simulink model "Group10_Pacemaker_FinalSimulink"  (R2020a)
settings: Solver=FixedStepAuto  StartTime=0.0  StopTime=300  FixedStep=1e-3  RelTol=1e-3  EnableMultiTasking=on
undefined symbols (not defined in the file): a, A0, A1, b, c, D0, D1, D10, D11, D12, D13, D2, D3, D4, D5, D6, D7, D8, D9, PTA0, PTA1, PTA2, PTB2, PTB23, PTB3, PTB9, PTC16, PTC17, PTC2, PTC3, PTC4, PTD0, PTD1, PTD2, PTD3
libraries: frdmk64flib x23, etargetslib x20, simulink x2, dspstat3 x1, hdlsllib x1
settings Model: ExtModeTrigDuration=5  Creator=jilsh  LastModifiedBy=Priya Patel
settings OptimizationCC: EnhancedBackFolding=on  PassReuseOutputArgsAs=Individual arguments  ZeroExternalMemoryAtStartup=off  ZeroInternalMemoryAtStartup=off  MaxStackSize=64  OptimizeBlockOrder=speed  DifferentSizesBufferReuse=on  OptimizationCustomize=off  EfficientTunableParamExpr=on
settings DebuggingCC: ParameterTunabilityLossMsg=error  SFMachineParentedDataDiag=error
settings HardwareCC: ProdBitPerPointer=32  ProdBitPerSizeT=32  ProdBitPerPtrDiffT=32  ProdLargestAtomicInteger=Long  ProdLargestAtomicFloat=Double  ProdWordSize=32  ProdHWDeviceType=ARM Compatible->ARM Cortex
settings SFSimCC: MATLABDynamicMemAlloc=off
settings RTWCC: SystemTargetFile=ert.tlc  HardwareBoard=NXP FRDM-K64F  TemplateMakefile=ert_default_tmf  Toolchain=GNU Tools for ARM Embedded Processors
settings CodeAppCC: ForceParamTrailComments=on  IgnoreCustomStorageClasses=off  OperatorAnnotations=on  SimulinkDataObjDesc=on  SFDataObjDesc=on  InsertBlockDesc=on
settings ERTTargetCC: ExtModeTransport=4  ExtModeMexFile=sendToCommService

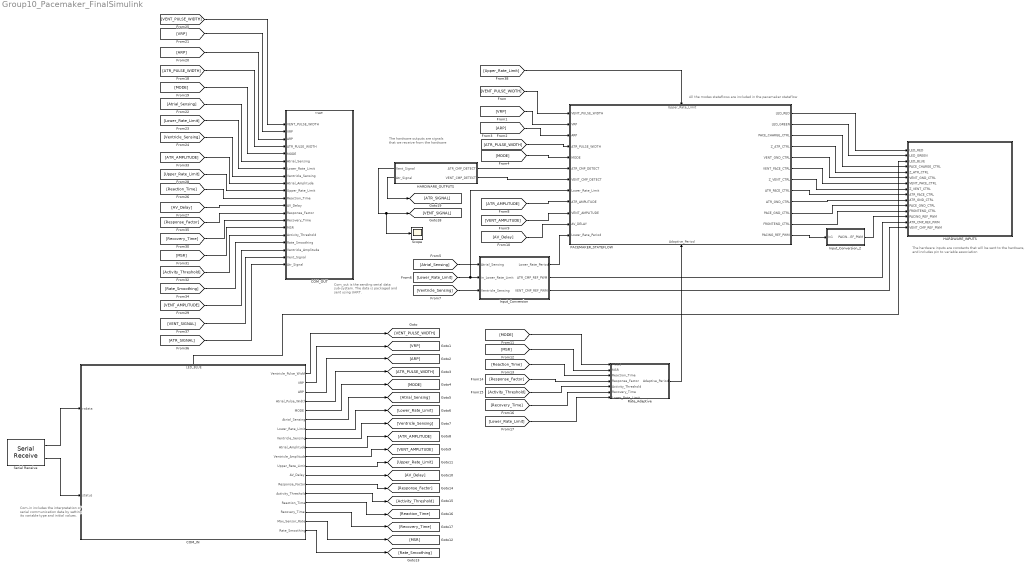
== system Group10_Pacemaker_FinalSimulink ==
  note: All the modes stateflows are included in the pacemaker stateflow
  note: The hardware inputs are constants that will be sent to the hardware, and includes pin to variable association
  note: The hardware outputs are signals
      |  that we receive from the hardware
  note: Com-in includes the interpretation of serial communication data by setting its variable type and initial values.
  note: Com_out is the sending serial data sub-system. The data is packaged and sent using UART.
  COM_IN : Stateflow chart  TreatAsAtomicUnit=on
      settings: PortSchema="{\"entries\":[{\"content\":{\"sides\":[{\"content\":{\"connectorIds\":[\"In1\",\"In2\"]},\"type\":\"ConnectorPlacement.EquallySpacedRectSide\",\"uuid\":\"1ea20d10-ec2b-4e93-9b01-0b71ee0000ee\"},{\"content\":{\"connectorIds\":[\"Out16\",\"Out17\",\"Out11\",\"Out2\",\"Out3\",\"Out10\",\"Out4\",\"Out5\",\"Out6\",\"Out7\",\"Out9\",\"Out12\",\"Out13\",\"Out18\",\"Out8\",\"Out14\",\"Out15\",\"Out19\"],\"side\":\"RIGHT\"},\"type\":\"ConnectorPlacement.EquallySpacedRectSide\",\"uuid\":\"2ad0043b-20de-4d86-8072-a48b2550d22e\"},{\"content\":{\"connectorIds\":[\"Out1\"],\"side\":\"TOP\"},\"type\":\"ConnectorPlacement.EquallySpacedRectSide\",\"uuid\":\"774fecc6-ead8-4e4a-b260-6b64e3396007\"},{\"content\":{\"connectorIds\":[],\"side\":\"BOTTOM\"},\"type\":\"ConnectorPlacement.EquallySpacedRectSide\",\"uuid\":\"8027b621-b96a-4f3b-ac6e-00bf94a638b1\"}]},\"type\":\"ConnectorPlacement.EquallySpacedConnector\",\"uuid\":\"2c430474-cea0-441a-a2e4-0cf18a0f8fb2\"}],\"packageUris\":[\"http://schema.mathworks.com/mf0/Connector/R2020b\"],\"version\":\"1.0\"}"
  COM_OUT : Subsystem
  HARDWARE_INPUTS : Subsystem
  HARDWARE_OUTPUTS : Subsystem
      settings: PortSchema="{\"entries\":[{\"content\":{\"sides\":[{\"content\":{\"connectorIds\":[\"Out3\",\"Out4\"]},\"type\":\"ConnectorPlacement.EquallySpacedRectSide\",\"uuid\":\"11d7f495-0e0c-41b1-9080-d2bc98e539d9\"},{\"content\":{\"connectorIds\":[\"Out1\",\"Out2\"],\"side\":\"RIGHT\"},\"type\":\"ConnectorPlacement.EquallySpacedRectSide\",\"uuid\":\"4942c8bf-5310-4876-b6bc-2d056dc4c66e\"},{\"content\":{\"connectorIds\":[],\"side\":\"TOP\"},\"type\":\"ConnectorPlacement.EquallySpacedRectSide\",\"uuid\":\"dbacaadd-fa2c-4803-9c39-533648a4c620\"}]},\"type\":\"ConnectorPlacement.EquallySpacedConnector\",\"uuid\":\"e98a59c8-405d-41a0-b96d-5878c2094b9d\"}],\"packageUris\":[\"http://schema.mathworks.com/mf0/Connector/R2020b\"],\"version\":\"1.0\"}"
  Input_Conversion : Subsystem
  Input_Conversion_2 : Subsystem
  PACEMAKER_STATEFLOW : Stateflow chart  TreatAsAtomicUnit=on
      settings: PortSchema="{\"entries\":[{\"content\":{\"sides\":[{\"content\":{\"connectorIds\":[\"In6\",\"In4\",\"In5\",\"In3\",\"In7\",\"In8\",\"In13\",\"In14\",\"In10\",\"In9\",\"In11\",\"In12\"]},\"type\":\"ConnectorPlacement.EquallySpacedRectSide\",\"uuid\":\"0c428793-4c7c-4531-b509-d420268b04c4\"},{\"content\":{\"connectorIds\":[\"Out1\",\"Out11\",\"Out2\",\"Out10\",\"Out4\",\"Out3\",\"Out9\",\"Out6\",\"Out8\",\"Out5\",\"Out7\",\"Out12\"],\"side\":\"RIGHT\"},\"type\":\"ConnectorPlacement.EquallySpacedRectSide\",\"uuid\":\"5c064d5f-3360-4ff7-b4a0-562d8799bc3d\"},{\"content\":{\"connectorIds\":[\"In1\"],\"side\":\"TOP\"},\"type\":\"ConnectorPlacement.EquallySpacedRectSide\",\"uuid\":\"3c80a0cf-2efb-4755-8997-5435fb1c804d\"},{\"content\":{\"connectorIds\":[\"In2\"],\"side\":\"BOTTOM\"},\"type\":\"ConnectorPlacement.EquallySpacedRectSide\",\"uuid\":\"a43fcd18-82d3-4111-8b38-3ebe4e29cce2\"}]},\"type\":\"ConnectorPlacement.EquallySpacedConnector\",\"uuid\":\"b1c06317-20b6-47a9-bece-373c8877e6e2\"}],\"packageUris\":[\"http://schema.mathworks.com/mf0/Connector/R2020b\"],\"version\":\"1.0\"}"
  Rate_Adaptive : Subsystem
  Scope : Scope
  Serial Receive : frdmk64flib/Serial Receive  SCIModule=0  Baudrate=uint32(9600)  Parity=None  StopBits=1  HardwareFlowControl=None  ByteOrder=LittleEndian  DataType=uint8  DataLength=52  BlockingMode=off  OutputStatus=on  SampleTime=-1
  wires:
  PACEMAKER_STATEFLOW/10(Z_ATR_CTRL) -> HARDWARE_INPUTS/5(Z_ATR_CTRL)
  PACEMAKER_STATEFLOW/4(VENT_GND_CTRL) -> HARDWARE_INPUTS/6(VENT_GND_CTRL)
  PACEMAKER_STATEFLOW/2(PACE_CHARGE_CTRL) -> HARDWARE_INPUTS/4(PACE_CHARGE_CTRL)
  PACEMAKER_STATEFLOW/3(VENT_PACE_CTRL) -> HARDWARE_INPUTS/7(VENT_PACE_CTRL)
  PACEMAKER_STATEFLOW/9(Z_VENT_CTRL) -> HARDWARE_INPUTS/8(Z_VENT_CTRL)
  PACEMAKER_STATEFLOW/8(ATR_GND_CTRL) -> HARDWARE_INPUTS/10(ATR_GND_CTRL)
  PACEMAKER_STATEFLOW/6(ATR_PACE_CTRL) -> HARDWARE_INPUTS/9(ATR_PACE_CTRL)
  PACEMAKER_STATEFLOW/5(PACE_GND_CTRL) -> HARDWARE_INPUTS/11(PACE_GND_CTRL)
  PACEMAKER_STATEFLOW/7(FRONTEND_CTRL) -> HARDWARE_INPUTS/12(FRONTEND_CTRL)
  HARDWARE_OUTPUTS/2(VENT_CMP_DETECT) -> PACEMAKER_STATEFLOW/13(VENT_CMP_DETECT)
  HARDWARE_OUTPUTS/1(ATR_CMP_DETECT) -> PACEMAKER_STATEFLOW/8(ATR_CMP_DETECT)
  Input_Conversion/2(ATR_CMP_REF_PWM) -> HARDWARE_INPUTS/14(ATR_CMP_REF_PWM)
  Input_Conversion/3(VENT_CMP_REF_PWM) -> HARDWARE_INPUTS/15(VENT_CMP_REF_PWM)
  PACEMAKER_STATEFLOW/11(LED_GREEN) -> HARDWARE_INPUTS/2(LED_GREEN)
  PACEMAKER_STATEFLOW/12(PACING_REF_PWM) -> Input_Conversion_2/1(In1)
  Input_Conversion_2/1(PACING_REF_PWM) -> HARDWARE_INPUTS/13(PACING_REF_PWM)
  [VENT_PULSE_WIDTH] -> PACEMAKER_STATEFLOW/6(VENT_PULSE_WIDTH)
  [VRP] -> PACEMAKER_STATEFLOW/4(VRP)
  [ARP] -> PACEMAKER_STATEFLOW/5(ARP)
  [ATR_PULSE_WIDTH] -> PACEMAKER_STATEFLOW/3(ATR_PULSE_WIDTH)
  [MODE] -> PACEMAKER_STATEFLOW/7(MODE)
  [Atrial_Sensing] -> Input_Conversion/1(Atrial_Sensing)
  [Lower_Rate_Limit] -> Input_Conversion/2(in_Lower_Rate_Limit), PACEMAKER_STATEFLOW/14(Lower_Rate_Limit)
  [Ventricle_Sensing] -> Input_Conversion/3(Ventricle_Sensing)
  [ATR_AMPLITUDE] -> PACEMAKER_STATEFLOW/10(ATR_AMPLITUDE)
  [VENT_AMPLITUDE] -> PACEMAKER_STATEFLOW/9(VENT_AMPLITUDE)
  [AV_Delay] -> PACEMAKER_STATEFLOW/11(AV_DELAY)
  [MODE] -> Rate_Adaptive/1(MODE)
  [MSR] -> Rate_Adaptive/2(MSR)
  [Reaction_Time] -> Rate_Adaptive/3(Reaction_Time)
  [Response_Factor] -> Rate_Adaptive/4(Response_Factor)
  [Activity_Threshold] -> Rate_Adaptive/5(Activity_Threshold)
  [Recovery_Time] -> Rate_Adaptive/6(Recovery_Time)
  [Lower_Rate_Limit] -> Rate_Adaptive/7(Lower_Rate_Limit)
  Rate_Adaptive/1(Adaptive_Period) -> PACEMAKER_STATEFLOW/2(Adaptive_Period)
  Serial Receive/2 -> COM_IN/2(status)
  Serial Receive/1 -> COM_IN/1(rxdata)
  COM_IN/16(Ventricle_Pulse_Width) -> [VENT_PULSE_WIDTH]
  COM_IN/17(VRP) -> [VRP]
  COM_IN/11(ARP) -> [ARP]
  COM_IN/2(Atrial_Pulse_Width) -> [ATR_PULSE_WIDTH]
  COM_IN/3(MODE) -> [MODE]
  COM_IN/10(Atrial_Sensing) -> [Atrial_Sensing]
  COM_IN/6(Atrial_Amplitude) -> [ATR_AMPLITUDE]
  COM_IN/7(Ventricle_Amplitude) -> [VENT_AMPLITUDE]
  COM_IN/5(Ventricle_Sensing) -> [Ventricle_Sensing]
  COM_IN/4(Lower_Rate_Limit) -> [Lower_Rate_Limit]
  COM_IN/9(Upper_Rate_Limit) -> [Upper_Rate_Limit]
  COM_IN/8(Reaction_Time) -> [Reaction_Time]
  COM_IN/12(AV_Delay) -> [AV_Delay]
  COM_IN/13(Response_Factor) -> [Response_Factor]
  COM_IN/14(Recovery_Time) -> [Recovery_Time]
  COM_IN/15(Max_Sensor_Rate) -> [MSR]
  COM_IN/18(Activity_Threshold) -> [Activity_Threshold]
  COM_IN/19(Rate_Smoothing) -> [Rate_Smoothing]
  [Ventricle_Sensing] -> COM_OUT/8(Ventricle_Sensing)
  [MSR] -> COM_OUT/15(MSR)
  [Rate_Smoothing] -> COM_OUT/17(Rate_Smoothing)
  [ARP] -> COM_OUT/3(ARP)
  [Response_Factor] -> COM_OUT/13(Response_Factor)
  [VRP] -> COM_OUT/2(VRP)
  [ATR_AMPLITUDE] -> COM_OUT/9(Atrial_Amplitude)
  [Activity_Threshold] -> COM_OUT/16(Activity_Threshold)
  [Reaction_Time] -> COM_OUT/11(Reaction_Time)
  [Recovery_Time] -> COM_OUT/14(Recovery_Time)
  [AV_Delay] -> COM_OUT/12(AV_Delay)
  [Lower_Rate_Limit] -> COM_OUT/7(Lower_Rate_Limit)
  [MODE] -> COM_OUT/5(MODE)
  [ATR_PULSE_WIDTH] -> COM_OUT/4(ATR_PULSE_WIDTH)
  [Upper_Rate_Limit] -> COM_OUT/10(Upper_Rate_Limit)
  [Atrial_Sensing] -> COM_OUT/6(Atrial_Sensing)
  [VENT_PULSE_WIDTH] -> COM_OUT/1(VENT_PULSE_WIDTH)
  PACEMAKER_STATEFLOW/1(LED_RED) -> HARDWARE_INPUTS/1(LED_RED)
  [VENT_AMPLITUDE] -> COM_OUT/18(Ventricle_Amplitude)
  HARDWARE_OUTPUTS/4(Atr_Signal) -> [ATR_SIGNAL]
  HARDWARE_OUTPUTS/3(Vent_Signal) -> Scope/1, [VENT_SIGNAL]
  [VENT_SIGNAL] -> COM_OUT/19(Vent_Signal)
  [ATR_SIGNAL] -> COM_OUT/20(Atr_Signal)
  Input_Conversion/1(Lower_Rate_Period) -> PACEMAKER_STATEFLOW/12(Lower_Rate_Period)
  COM_IN/1(LED_BLUE) -> HARDWARE_INPUTS/3(LED_BLUE)
  [Upper_Rate_Limit] -> PACEMAKER_STATEFLOW/1(Upper_Rate_Limit)

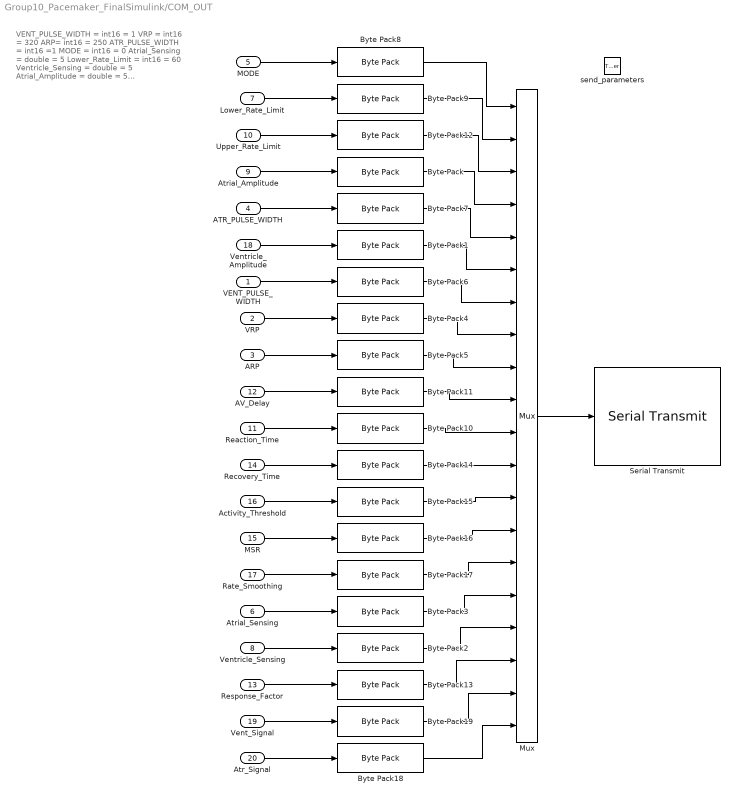
== system Group10_Pacemaker_FinalSimulink/COM_OUT ==
  note: VENT_PULSE_WIDTH = int16 = 1
      | VRP = int16 = 320
      | ARP= int16 = 250
      | ATR_PULSE_WIDTH = int16 =1
      | MODE =  int16 = 0
      | Atrial_Sensing = double = 5
      | Lower_Rate_Limit = int16 = 60
      | Ventricle_Sensing = double = 5
      | Atrial_Amplitude = double = 5
      | Ventricle_Amplitude = double = 5
      | Upper Rate Limit = int16 =120
      | Reaction_Time = int16 = 30
      | AV_Delay = int16 = 100
      | Response_Factor = in16 =8
      | Recovery_Time =int16 =5
      | MSR = int16 =120
      | Activity_Threshold = int16 = 1
      | Rate Smoothening = int16 = 0
  VENT_PULSE_WIDTH : Inport
  VRP : Inport  Port=2
  ARP : Inport  Port=3
  ATR_PULSE_WIDTH : Inport  Port=4
  MODE : Inport  Port=5
  Atrial_Sensing : Inport  Port=6
  Lower_Rate_Limit : Inport  Port=7
  Ventricle_Sensing : Inport  Port=8
  Atrial_Amplitude : Inport  Port=9
  Upper_Rate_Limit : Inport  Port=10
  Reaction_Time : Inport  Port=11
  AV_Delay : Inport  Port=12
  Response_Factor : Inport  Port=13
  Recovery_Time : Inport  Port=14
  MSR : Inport  Port=15
  Activity_Threshold : Inport  Port=16
  Rate_Smoothing : Inport  Port=17
  Ventricle_Amplitude : Inport  Port=18
  Vent_Signal : Inport  Port=19
  Atr_Signal : Inport  Port=20
  send_parameters : TriggerPort  TriggerType=function-call  IsSimulinkFunction=on  FunctionName=send_parameters  VariantControl=(inherit)  PortDimensions=1
  Byte Pack{,1..3} (4 alike) : etargetslib/Byte Pack  datatypes={'single'}  byteAlign=1
  Byte Pack{4..14,16..17} (13 alike) : etargetslib/Byte Pack  datatypes={'uint16'}  byteAlign=1
  Byte Pack15 : etargetslib/Byte Pack  datatypes={'double'}  byteAlign=1
  Byte Pack18 : etargetslib/Byte Pack  datatypes={'double'}  byteAlign=1
  Byte Pack19 : etargetslib/Byte Pack  datatypes={'double'}  byteAlign=1
  Mux : Mux  Inputs=20
  Serial Transmit : frdmk64flib/Serial Transmit  SCIModule=0  Baudrate=uint32(9600)  Parity=None  StopBits=1  HardwareFlowControl=None  ByteOrder=LittleEndian  BlockingMode=on  OutputStatus=off
  wires:
  Mux/1 -> Serial Transmit/1
  Atrial_Sensing/1 -> Byte Pack3/1
  VENT_PULSE_WIDTH/1 -> Byte Pack6/1
  VRP/1 -> Byte Pack4/1
  ARP/1 -> Byte Pack5/1
  ATR_PULSE_WIDTH/1 -> Byte Pack7/1
  MODE/1 -> Byte Pack8/1
  Lower_Rate_Limit/1 -> Byte Pack9/1
  Ventricle_Sensing/1 -> Byte Pack2/1
  Atrial_Amplitude/1 -> Byte Pack/1
  Ventricle_Amplitude/1 -> Byte Pack1/1
  Upper_Rate_Limit/1 -> Byte Pack12/1
  Reaction_Time/1 -> Byte Pack10/1
  AV_Delay/1 -> Byte Pack11/1
  Response_Factor/1 -> Byte Pack13/1
  Recovery_Time/1 -> Byte Pack14/1
  Activity_Threshold/1 -> Byte Pack15/1
  MSR/1 -> Byte Pack16/1
  Rate_Smoothing/1 -> Byte Pack17/1
  Byte Pack8/1 -> Mux/1
  Byte Pack9/1 -> Mux/2
  Byte Pack12/1 -> Mux/3
  Byte Pack/1 -> Mux/4
  Byte Pack1/1 -> Mux/6
  Byte Pack7/1 -> Mux/5
  Byte Pack6/1 -> Mux/7
  Byte Pack5/1 -> Mux/9
  Byte Pack4/1 -> Mux/8
  Byte Pack11/1 -> Mux/10
  Byte Pack10/1 -> Mux/11
  Byte Pack14/1 -> Mux/12
  Byte Pack15/1 -> Mux/13
  Byte Pack16/1 -> Mux/14
  Byte Pack17/1 -> Mux/15
  Byte Pack3/1 -> Mux/16
  Byte Pack2/1 -> Mux/17
  Byte Pack13/1 -> Mux/18
  Vent_Signal/1 -> Byte Pack19/1
  Atr_Signal/1 -> Byte Pack18/1
  Byte Pack19/1 -> Mux/19
  Byte Pack18/1 -> Mux/20

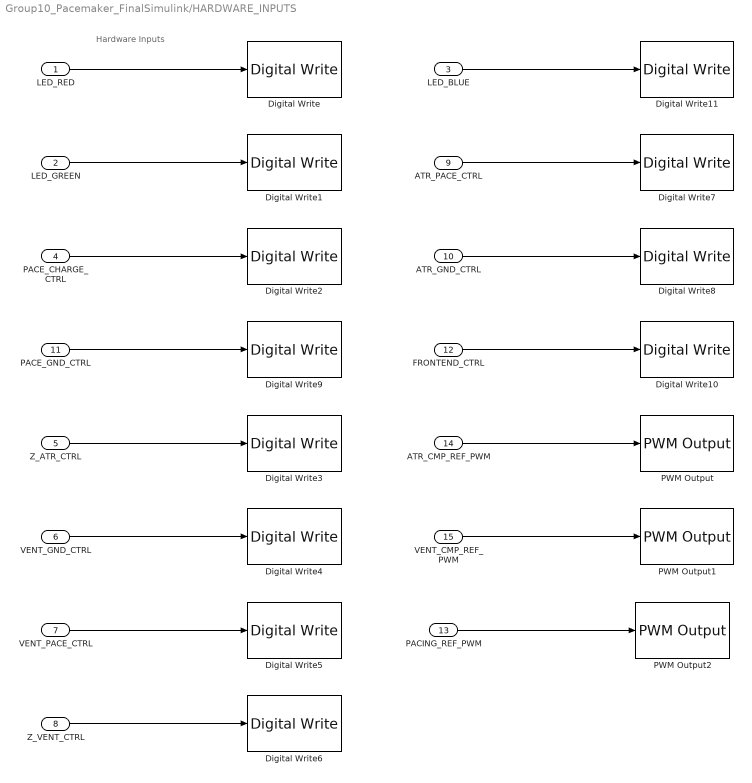
== system Group10_Pacemaker_FinalSimulink/HARDWARE_INPUTS ==
  note: Hardware Inputs
  LED_RED : Inport  OutDataTypeStr=boolean
  LED_GREEN : Inport  Port=2  OutDataTypeStr=boolean
  LED_BLUE : Inport  Port=3  OutDataTypeStr=boolean
  PACE_CHARGE_CTRL : Inport  Port=4  OutDataTypeStr=boolean
  Z_ATR_CTRL : Inport  Port=5  OutDataTypeStr=boolean
  VENT_GND_CTRL : Inport  Port=6  OutDataTypeStr=boolean
  VENT_PACE_CTRL : Inport  Port=7  OutDataTypeStr=boolean
  Z_VENT_CTRL : Inport  Port=8  OutDataTypeStr=boolean
  ATR_PACE_CTRL : Inport  Port=9  OutDataTypeStr=boolean
  ATR_GND_CTRL : Inport  Port=10  OutDataTypeStr=boolean
  PACE_GND_CTRL : Inport  Port=11  OutDataTypeStr=boolean
  FRONTEND_CTRL : Inport  Port=12  OutDataTypeStr=boolean
  PACING_REF_PWM : Inport  Port=13
  ATR_CMP_REF_PWM : Inport  Port=14
  VENT_CMP_REF_PWM : Inport  Port=15
  Digital Write : frdmk64flib/Digital Write  Whichpin=RED_LED
  Digital Write1 : frdmk64flib/Digital Write  Whichpin=GREEN_LED
  Digital Write10 : frdmk64flib/Digital Write  Whichpin=PTD1 (D13)
  Digital Write11 : frdmk64flib/Digital Write  Whichpin=BLUE_LED
  Digital Write2 : frdmk64flib/Digital Write  Whichpin=PTB9 (D2)
  Digital Write3 : frdmk64flib/Digital Write  Whichpin=PTB23 (D4)
  Digital Write4 : frdmk64flib/Digital Write  Whichpin=PTD3 (D12)
  Digital Write5 : frdmk64flib/Digital Write  Whichpin=PTC4 (D9)
  Digital Write6 : frdmk64flib/Digital Write  Whichpin=PTC3 (D7)
  Digital Write7 : frdmk64flib/Digital Write  Whichpin=PTA0 (D8)
  Digital Write8 : frdmk64flib/Digital Write  Whichpin=PTD2 (D11)
  Digital Write9 : frdmk64flib/Digital Write  Whichpin=PTD0 (D10)
  PWM Output : frdmk64flib/PWM Output  Whichpin=PTC2 (D6)  InitialFrequency=2000  InitialDutyCycle=0
  PWM Output1 : frdmk64flib/PWM Output  Whichpin=PTA1 (D3)  InitialFrequency=2000  InitialDutyCycle=0
  PWM Output2 : frdmk64flib/PWM Output  Whichpin=PTA2 (D5)  InitialFrequency=2000  InitialDutyCycle=0
  wires:
  LED_RED/1 -> Digital Write/1
  LED_GREEN/1 -> Digital Write1/1
  Z_ATR_CTRL/1 -> Digital Write3/1
  VENT_GND_CTRL/1 -> Digital Write4/1
  VENT_PACE_CTRL/1 -> Digital Write5/1
  ATR_GND_CTRL/1 -> Digital Write8/1
  ATR_PACE_CTRL/1 -> Digital Write7/1
  Z_VENT_CTRL/1 -> Digital Write6/1
  PACE_GND_CTRL/1 -> Digital Write9/1
  FRONTEND_CTRL/1 -> Digital Write10/1
  ATR_CMP_REF_PWM/1 -> PWM Output/1
  VENT_CMP_REF_PWM/1 -> PWM Output1/1
  PACING_REF_PWM/1 -> PWM Output2/1
  PACE_CHARGE_CTRL/1 -> Digital Write2/1
  LED_BLUE/1 -> Digital Write11/1

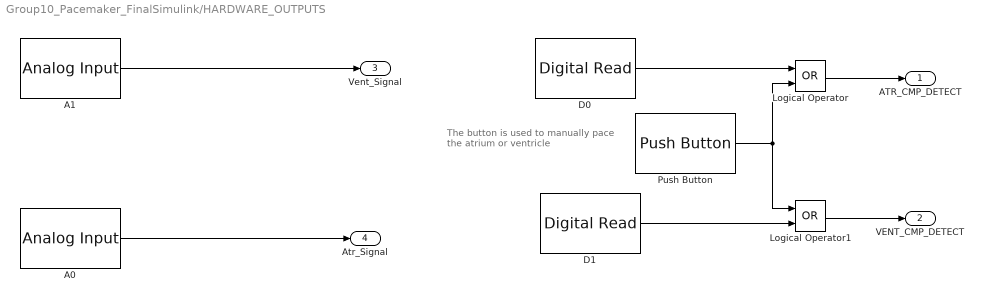
== system Group10_Pacemaker_FinalSimulink/HARDWARE_OUTPUTS ==
  note: The button is used to manually pace
      | the atrium or ventricle
  A0 : frdmk64flib/Analog Input  Whichpin=PTB2 (A0)  SampleTime=-1
  A1 : frdmk64flib/Analog Input  Whichpin=PTB3 (A1)  SampleTime=-1
  D0 : frdmk64flib/Digital Read  Whichpin=PTC16 (D0)  SampleTime=-1
  D1 : frdmk64flib/Digital Read  Whichpin=PTC17 (D1)  SampleTime=-1
  Logical Operator : Logic  Operator=OR  AllPortsSameDT=off
  Logical Operator1 : Logic  Operator=OR  AllPortsSameDT=off
  Push Button : frdmk64flib/Push Button  Whichswitch=SW2  SampleTime1=-1
  ATR_CMP_DETECT : Outport  OutDataTypeStr=boolean
  VENT_CMP_DETECT : Outport  Port=2  OutDataTypeStr=boolean
  Vent_Signal : Outport  Port=3
  Atr_Signal : Outport  Port=4
  wires:
  D0/1 -> Logical Operator/1
  D1/1 -> Logical Operator1/2
  Push Button/1 -> Logical Operator1/1, Logical Operator/2
  Logical Operator/1 -> ATR_CMP_DETECT/1
  Logical Operator1/1 -> VENT_CMP_DETECT/1
  A0/1 -> Atr_Signal/1
  A1/1 -> Vent_Signal/1

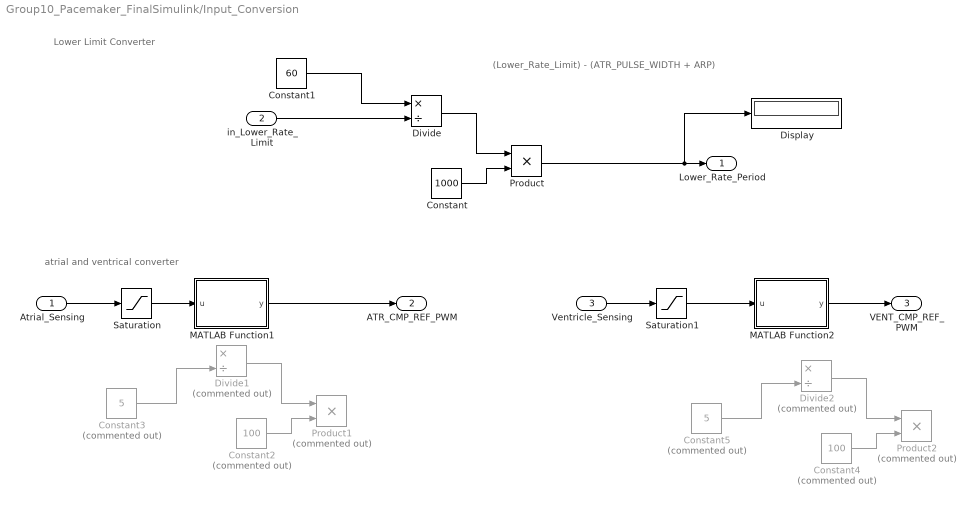
== system Group10_Pacemaker_FinalSimulink/Input_Conversion ==
  note: (Lower_Rate_Limit) - (ATR_PULSE_WIDTH + ARP)
  note: atrial and ventrical converter
  note: Lower Limit Converter
  Atrial_Sensing : Inport
  in_Lower_Rate_Limit : Inport  Port=2  OutDataTypeStr=uint16
  Ventricle_Sensing : Inport  Port=3
  Constant : Constant  Value=1000  OutDataTypeStr=double
  Constant1 : Constant  Value=60  OutDataTypeStr=double
  Constant2 : Constant  Commented=on  Value=100  OutDataTypeStr=int16
  Constant3 : Constant  Commented=on  Value=5  OutDataTypeStr=int16
  Constant4 : Constant  Commented=on  Value=100  VectorParams1D=off  OutDataTypeStr=int16
  Constant5 : Constant  Commented=on  Value=5  OutDataTypeStr=int16
  Display : Display
  Divide : Product  Inputs=*/  OutDataTypeStr=double
  Divide1 : Product  Commented=on  Inputs=*/  OutDataTypeStr=double
  Divide2 : Product  Commented=on  Inputs=*/  OutDataTypeStr=double
  MATLAB Function1 : MATLAB Function  TreatAsAtomicUnit=on
  MATLAB Function2 : MATLAB Function  TreatAsAtomicUnit=on
  Product : Product  OutDataTypeStr=double
  Product1 : Product  Commented=on  OutDataTypeStr=int16
  Product2 : Product  Commented=on  OutDataTypeStr=int16
  Saturation : Saturate  UpperLimit=4  LowerLimit=0.65  LinearizeAsGain=off  OutDataTypeStr=double
  Saturation1 : Saturate  UpperLimit=4  LowerLimit=0.65  OutDataTypeStr=double
  Lower_Rate_Period : Outport  OutDataTypeStr=double
  ATR_CMP_REF_PWM : Outport  Port=2
  VENT_CMP_REF_PWM : Outport  Port=3
  wires:
  Atrial_Sensing/1 -> Saturation/1
  Ventricle_Sensing/1 -> Saturation1/1
  Constant2/1 -> Product1/2
  Divide1/1 -> Product1/1
  Constant3/1 -> Divide1/2
  Saturation1/1 -> MATLAB Function2/1(u)
  Constant4/1 -> Product2/2
  Divide2/1 -> Product2/1
  Constant5/1 -> Divide2/2
  MATLAB Function2/1(y) -> VENT_CMP_REF_PWM/1
  Saturation/1 -> MATLAB Function1/1(u)
  MATLAB Function1/1(y) -> ATR_CMP_REF_PWM/1
  Constant1/1 -> Divide/1
  in_Lower_Rate_Limit/1 -> Divide/2
  Divide/1 -> Product/1
  Constant/1 -> Product/2
  Product/1 -> Display/1, Lower_Rate_Period/1

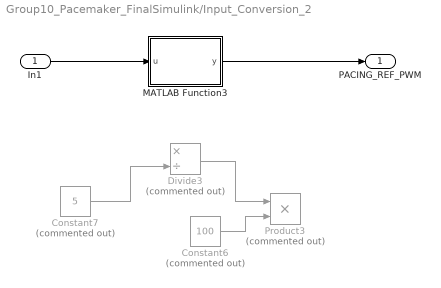
== system Group10_Pacemaker_FinalSimulink/Input_Conversion_2 ==
  In1 : Inport
  Constant6 : Constant  Commented=on  Value=100  VectorParams1D=off  OutDataTypeStr=int16
  Constant7 : Constant  Commented=on  Value=5  OutDataTypeStr=int16
  Divide3 : Product  Commented=on  Inputs=*/  OutDataTypeStr=double
  MATLAB Function3 : MATLAB Function  TreatAsAtomicUnit=on
  Product3 : Product  Commented=on  OutDataTypeStr=int16
  PACING_REF_PWM : Outport
  wires:
  Constant7/1 -> Divide3/2
  In1/1 -> MATLAB Function3/1(u)
  Divide3/1 -> Product3/1
  Constant6/1 -> Product3/2
  MATLAB Function3/1(y) -> PACING_REF_PWM/1

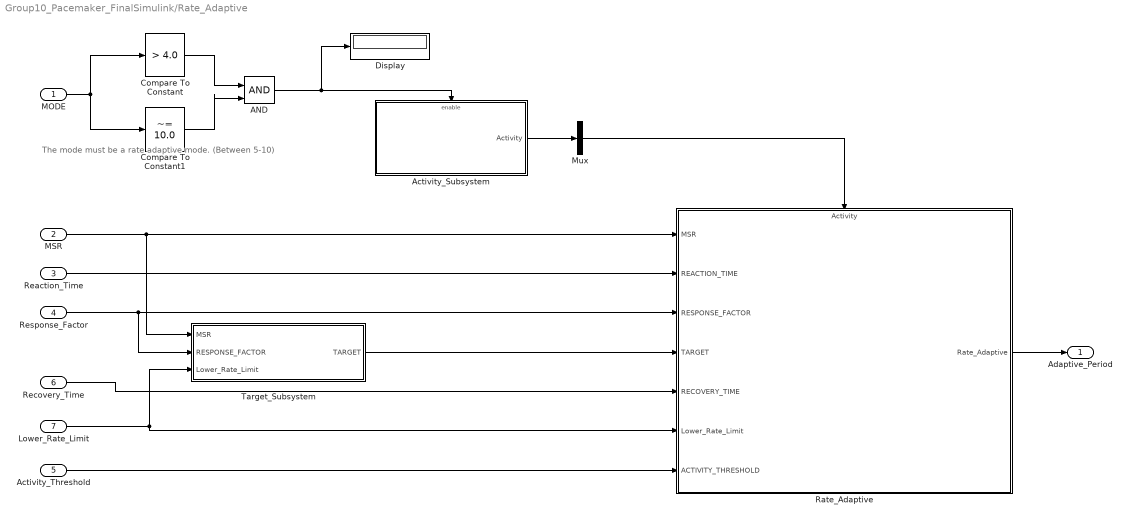
== system Group10_Pacemaker_FinalSimulink/Rate_Adaptive ==
  note: The mode must be a rate adaptive mode. (Between 5-10)
  MODE : Inport  OutDataTypeStr=uint16
  MSR : Inport  Port=2  OutDataTypeStr=uint16
  Reaction_Time : Inport  Port=3  OutDataTypeStr=uint16
  Response_Factor : Inport  Port=4  OutDataTypeStr=uint16
  Activity_Threshold : Inport  Port=5  OutDataTypeStr=double
  Recovery_Time : Inport  Port=6  OutDataTypeStr=uint16
  Lower_Rate_Limit : Inport  Port=7  OutDataTypeStr=uint16
  AND : Logic  IconShape=distinctive  AllPortsSameDT=off  OutDataTypeStr=boolean
  Activity_Subsystem : Subsystem
  Compare To Constant : simulink/Logic and Bit Operations/Compare To Constant  relop=>  const=4.0  OutDataTypeStr=boolean
  Compare To Constant1 : simulink/Logic and Bit Operations/Compare To Constant  relop=~=  const=10.0  OutDataTypeStr=boolean
  Display : Display
  Mux : Mux  Inputs=1
  Rate_Adaptive : Subsystem
      settings: PortSchema="{\"entries\":[{\"content\":{\"sides\":[{\"content\":{\"connectorIds\":[\"In1\",\"In2\",\"In3\",\"In4\",\"In5\",\"In6\",\"In7\"]},\"type\":\"ConnectorPlacement.EquallySpacedRectSide\",\"uuid\":\"ecef5992-6168-4615-8079-152f4001d897\"},{\"content\":{\"connectorIds\":[\"Out1\"],\"side\":\"RIGHT\"},\"type\":\"ConnectorPlacement.EquallySpacedRectSide\",\"uuid\":\"4b0443a4-3c4f-432b-8acf-b8853e3911f3\"},{\"content\":{\"connectorIds\":[\"In8\"],\"side\":\"TOP\"},\"type\":\"ConnectorPlacement.EquallySpacedRectSide\",\"uuid\":\"9eb25122-da38-4088-8f00-2d2dff5efbee\"},{\"content\":{\"connectorIds\":[],\"side\":\"BOTTOM\"},\"type\":\"ConnectorPlacement.EquallySpacedRectSide\",\"uuid\":\"f562ad64-64af-4bdb-b61f-82ac1a60a400\"}]},\"type\":\"ConnectorPlacement.EquallySpacedConnector\",\"uuid\":\"02b21474-b9be-4120-8392-47ed1544c592\"}],\"packageUris\":[\"http://schema.mathworks.com/mf0/Connector/R2020b\"],\"version\":\"1.0\"}"
  Target_Subsystem : Subsystem
  Adaptive_Period : Outport  OutDataTypeStr=uint16
  wires:
  MODE/1 -> Compare To Constant1/1, Compare To Constant/1
  Compare To Constant/1 -> AND/1
  Compare To Constant1/1 -> AND/2
  AND/1 -> Display/1, Activity_Subsystem/Enable
  Activity_Subsystem/1(Activity) -> Mux/1
  Response_Factor/1 -> Rate_Adaptive/3(RESPONSE_FACTOR), Target_Subsystem/2(RESPONSE_FACTOR)
  Lower_Rate_Limit/1 -> Rate_Adaptive/6(Lower_Rate_Limit), Target_Subsystem/3(Lower_Rate_Limit)
  Activity_Threshold/1 -> Rate_Adaptive/7(ACTIVITY_THRESHOLD)
  Mux/1 -> Rate_Adaptive/8(Activity)
  MSR/1 -> Target_Subsystem/1(MSR), Rate_Adaptive/1(MSR)
  Reaction_Time/1 -> Rate_Adaptive/2(REACTION_TIME)
  Target_Subsystem/1(TARGET) -> Rate_Adaptive/4(TARGET)
  Recovery_Time/1 -> Rate_Adaptive/5(RECOVERY_TIME)
  Rate_Adaptive/1(Rate_Adaptive) -> Adaptive_Period/1

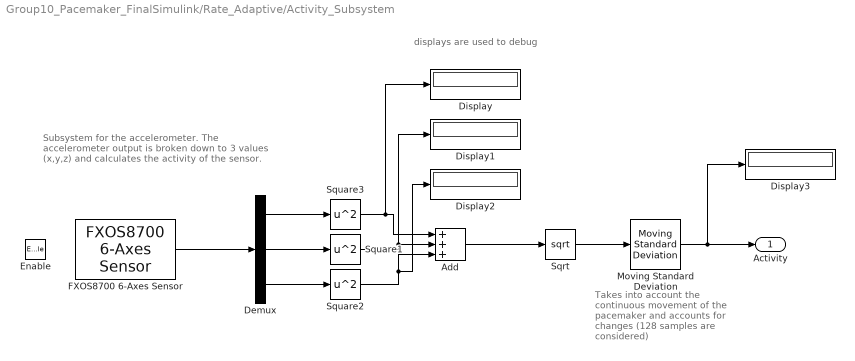
== system Group10_Pacemaker_FinalSimulink/Rate_Adaptive/Activity_Subsystem ==
  note: displays are used to debug
  note: Takes into account the continuous movement of the pacemaker and accounts for changes (128 samples are considered)
  note: Subsystem for the accelerometer.
      | The accelerometer output is broken down to
      | 3 values (x,y,z) and calculates the activity of the sensor.
  Enable : EnablePort
  Add : Sum  Inputs=+++
  Demux : Demux  Outputs=3
  Display{,1..3} (4 alike) : Display
  FXOS8700 6-Axes Sensor : frdmk64flib/FXOS8700 6-Axes Sensor  Activesensor=Accelerometer only  ODR=800Hz  HybridODR=400Hz  Accelfullrange=-4g to +4g  SampleTime=-1
  Moving Standard Deviation : dspstat3/Moving Standard Deviation  Method=Sliding window  ForgettingFactorPort=off  SpecifyWindowLength=on  WindowLength=128  ForgettingFactor=0.9  SimulateUsing=Code generation
      settings: SourceProductBaseCode=DS
  Sqrt : Sqrt  SaturateOnIntegerOverflow=on
  Square1 : Math  Operator=square  OutDataTypeStr=double  SaturateOnIntegerOverflow=on
  Square2 : Math  Operator=square  OutDataTypeStr=double  SaturateOnIntegerOverflow=on
  Square3 : Math  Operator=square  OutDataTypeStr=double  SaturateOnIntegerOverflow=on
  Activity : Outport
  wires:
  FXOS8700 6-Axes Sensor/1 -> Demux/1
  Demux/3 -> Square2/1
  Square1/1 -> Display1/1, Add/2
  Add/1 -> Sqrt/1
  Demux/2 -> Square1/1
  Square3/1 -> Display/1, Add/1
  Square2/1 -> Display2/1, Add/3
  Demux/1 -> Square3/1
  Sqrt/1 -> Moving Standard Deviation/1
  Moving Standard Deviation/1 -> Display3/1, Activity/1

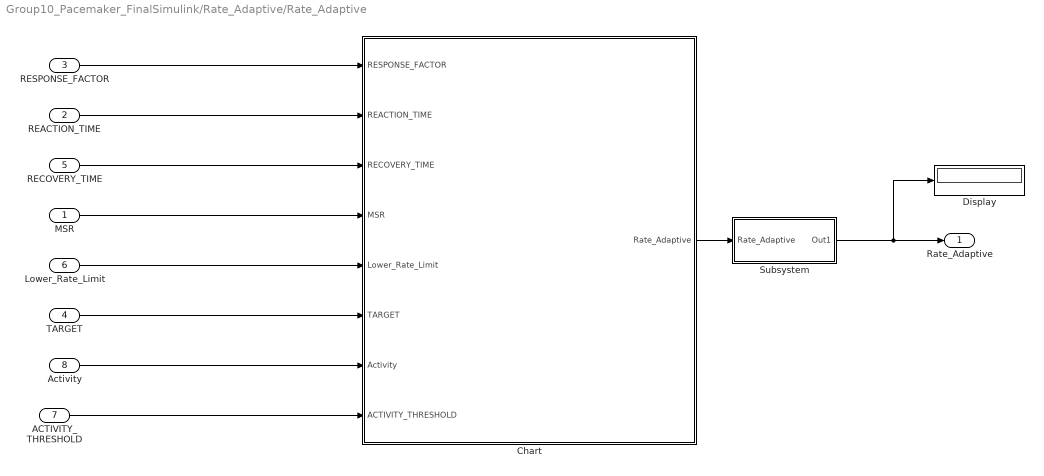
== system Group10_Pacemaker_FinalSimulink/Rate_Adaptive/Rate_Adaptive ==
  MSR : Inport
  REACTION_TIME : Inport  Port=2
  RESPONSE_FACTOR : Inport  Port=3
  TARGET : Inport  Port=4
  RECOVERY_TIME : Inport  Port=5
  Lower_Rate_Limit : Inport  Port=6
  ACTIVITY_THRESHOLD : Inport  Port=7  OutDataTypeStr=double
  Activity : Inport  Port=8
  Chart : Stateflow chart  TreatAsAtomicUnit=on
  Display : Display
  Subsystem : Subsystem
  Rate_Adaptive : Outport
  wires:
  RESPONSE_FACTOR/1 -> Chart/1(RESPONSE_FACTOR)
  REACTION_TIME/1 -> Chart/2(REACTION_TIME)
  RECOVERY_TIME/1 -> Chart/3(RECOVERY_TIME)
  ACTIVITY_THRESHOLD/1 -> Chart/8(ACTIVITY_THRESHOLD)
  MSR/1 -> Chart/4(MSR)
  Lower_Rate_Limit/1 -> Chart/5(Lower_Rate_Limit)
  TARGET/1 -> Chart/6(TARGET)
  Activity/1 -> Chart/7(Activity)
  Chart/1(Rate_Adaptive) -> Subsystem/1(Rate_Adaptive)
  Subsystem/1(Out1) -> Display/1, Rate_Adaptive/1

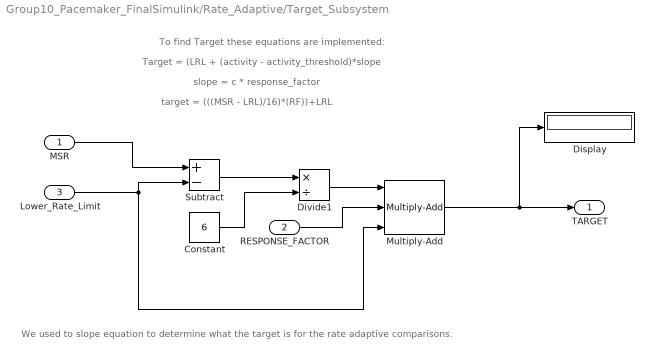
== system Group10_Pacemaker_FinalSimulink/Rate_Adaptive/Target_Subsystem ==
  note: target = (((MSR - LRL)/16)*(RF))+LRL
  note: We used to slope equation to determine what the target is for the rate adaptive comparisons.
  note: slope = c * response_factor
  note: Target = (LRL + (activity - activity_threshold)*slope
  note: To find Target these equations are implemented:
  MSR : Inport
  RESPONSE_FACTOR : Inport  Port=2
  Lower_Rate_Limit : Inport  Port=3
  Constant : Constant  Value=6
  Display : Display
  Divide1 : Product  Inputs=*/
  Multiply-Add : hdlsllib/HDL Operations/Multiply-Add  Function=c+(a.*b)  datatype=uint16  RndMeth=Round  DoSatur=off  FMA=off
      settings: SourceProductBaseCode=SL
  Subtract : Sum  Inputs=+-
  TARGET : Outport  OutDataTypeStr=uint16
  wires:
  RESPONSE_FACTOR/1 -> Multiply-Add/2
  Constant/1 -> Divide1/2
  MSR/1 -> Subtract/1
  Lower_Rate_Limit/1 -> Subtract/2, Multiply-Add/3
  Divide1/1 -> Multiply-Add/1
  Multiply-Add/1 -> Display/1, TARGET/1
  Subtract/1 -> Divide1/1

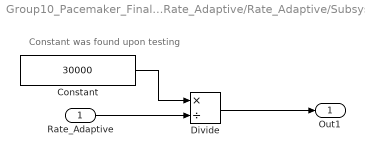
== system Group10_Pacemaker_FinalSimulink/Rate_Adaptive/Rate_Adaptive/Subsystem ==
  note: Constant was found upon testing
  Rate_Adaptive : Inport
  Constant : Constant  Value=30000  OutDataTypeStr=uint16
  Divide : Product  Inputs=*/
  Out1 : Outport  OutDataTypeStr=uint16
  wires:
  Constant/1 -> Divide/1
  Rate_Adaptive/1 -> Divide/2
  Divide/1 -> Out1/1

== matlab function Group10_Pacemaker_FinalSimulink/Input_Conversion_2/MATLAB Function3 ==
  data: u input; y output
function y = fcn(u)

y = u./5.*100;

== stateflow chart Group10_Pacemaker_FinalSimulink/Rate_Adaptive/Rate_Adaptive/Chart ==
  note: The step up and step down variables are finding the step sizes in order to reach the target rate
  state State1
    entry:
    Rate_Adaptive = Lower_Rate_Limit;
    %when activity is less than activity threshold the rate adaptive is equal to LRL
  state State3
    entry:
    Rate_Adaptive = TARGET;
    %If activity is continued then the rate adaptive will eventually reach the target rate
  state State2
    entry:
    Rate_Adaptive = Rate_Adaptive + Step_Up;
    %Rate adaptive is calculated using step size when activity is high
  state State5
    entry:
    Rate_Adaptive = Rate_Adaptive - Step_Down;
    %continue to decrease rate adaptive until LRL is reached
  state State4
    entry:
    Rate_Adaptive = Rate_Adaptive - Step_Up;
    %once the activty starts decreasing we need to decrease rate adaptive
  (default) -> State1 : {Step_Up = ceil((TARGET - Lower_Rate_Limit)/REACTION_TIME);
      | Step_Down = ceil((TARGET - Lower_Rate_Limit)/RECOVERY_TIME)}
  State1 -> State1 [order 1] : [Activity < ACTIVITY_THRESHOLD]
  State2 -> State2 [order 2] : after(1000,msec)[Rate_Adaptive <= TARGET]
  State3 -> State3 [order 2] : [Activity > ACTIVITY_THRESHOLD]
  State1 -> State2 [order 2] : [Activity >= ACTIVITY_THRESHOLD]
  State2 -> State3 [order 3] : [Rate_Adaptive >= TARGET]
  State3 -> State5 [order 1] : [Activity < ACTIVITY_THRESHOLD]
  State5 -> State1 [order 1] : [Rate_Adaptive <= Lower_Rate_Limit]
  State5 -> State2 [order 3] : [Activity >= ACTIVITY_THRESHOLD]
  State2 -> State4 [order 1] : [Activity < ACTIVITY_THRESHOLD]
  State4 -> State2 [order 1] : [Activity >= ACTIVITY_THRESHOLD]
  State4 -> State5 [order 2] : [after(1000,msec)]
  State5 -> State5 [order 2] : after(1000,msec)[Rate_Adaptive >= Lower_Rate_Limit]
  data: RESPONSE_FACTOR input; REACTION_TIME input; RECOVERY_TIME input; MSR input; Lower_Rate_Limit input; TARGET input; Activity input; ACTIVITY_THRESHOLD input; Rate_Adaptive output; Step_Up local uint16; Step_Down local uint16

== stateflow chart Group10_Pacemaker_FinalSimulink/PACEMAKER_STATEFLOW ==
  state AAIR_VVIR
    state AAIR_CHARGING
      entry:
      FRONTEND_CTRL = true;
      PACE_GND_CTRL = true;
      VENT_PACE_CTRL=false;
      ATR_PACE_CTRL=false;
      PACE_CHARGE_CTRL=true;
      ATR_GND_CTRL=false;
      VENT_GND_CTRL=true;
      LED_RED = false;
      PACING_REF_PWM = ATR_AMPLITUDE;
      % charging and discharging the capacitors
      % setting the pacing pwm to Atrium Amplitude
    state VVI_CHARGING
      entry:
      FRONTEND_CTRL = true;
      PACE_GND_CTRL = true;
      VENT_PACE_CTRL=false;
      ATR_PACE_CTRL=false;
      PACE_CHARGE_CTRL=true;
      ATR_GND_CTRL=false;
      VENT_GND_CTRL=true;
      LED_GREEN = false;
      PACING_REF_PWM = VENT_AMPLITUDE;
      % charging and discharging the capacitors
      % setting the pacing pwm to Atrium Amplitude
    state VVI_ATRIAL_PACING
      entry:
      FRONTEND_CTRL = false;
      PACE_GND_CTRL = true;
      VENT_PACE_CTRL=true;
      ATR_PACE_CTRL=false;
      PACE_CHARGE_CTRL=false;
      ATR_GND_CTRL=false;
      VENT_GND_CTRL=false;
      LED_GREEN = true;
      % pacemaker will respond by sending a signal
    state AAI_ATRIAL_PACING
      entry:
      FRONTEND_CTRL = false;
      PACE_GND_CTRL = true;
      VENT_PACE_CTRL=false;
      ATR_PACE_CTRL=true;
      PACE_CHARGE_CTRL=false;
      ATR_GND_CTRL=false;
      VENT_GND_CTRL=false;
      LED_RED = true;
      % pacemaker will respond by sending a signal
    state AAI_ARP_STATE
      entry:
      PACE_GND_CTRL = true;
      VENT_PACE_CTRL=false;
      ATR_PACE_CTRL=false;
      PACE_CHARGE_CTRL=true;
      ATR_GND_CTRL=true;
      VENT_GND_CTRL=false;
      LED_RED= false;
      PACING_REF_PWM = ATR_AMPLITUDE;
      % enters this state when a atrial signal is detected
    state VVI_VRP_STATE
      entry:
      PACE_GND_CTRL = true;
      VENT_PACE_CTRL=false;
      ATR_PACE_CTRL=false;
      PACE_CHARGE_CTRL=true;
      ATR_GND_CTRL=false;
      VENT_GND_CTRL=true;
      LED_GREEN = false;
      % enters this state when a Ventricular signal is detected
    AAIR_CHARGING -> AAIR_VVIR [order 2] : [MODE ~= 7]
    AAIR_VVIR.VVI_CHARGING -> AAIR_VVIR [order 2] : [MODE~=8]
    (default) -> (junction 162)
    (junction 162) -> AAIR_VVIR.VVI_CHARGING [order 2]
    (junction 162) -> AAIR_CHARGING [order 1] : [MODE == 7]
    AAIR_VVIR.VVI_CHARGING -> AAIR_VVIR.VVI_ATRIAL_PACING [order 1] : after(Adaptive_Period - VENT_PULSE_WIDTH-VRP, msec)
    AAIR_CHARGING -> AAIR_VVIR.AAI_ATRIAL_PACING [order 1] : after(Adaptive_Period - ATR_PULSE_WIDTH - ARP, msec)
    AAIR_VVIR.VVI_VRP_STATE -> AAIR_VVIR.VVI_CHARGING : after(VRP, msec)
    AAIR_VVIR.VVI_CHARGING -> AAIR_VVIR.VVI_VRP_STATE [order 3] : [VENT_CMP_DETECT == true]
    AAIR_CHARGING -> AAIR_VVIR.AAI_ARP_STATE [order 3] : [ATR_CMP_DETECT == true]
    AAIR_VVIR.AAI_ARP_STATE -> AAIR_CHARGING : after(ARP, msec)
    AAIR_VVIR.VVI_ATRIAL_PACING -> AAIR_VVIR.VVI_VRP_STATE : after(VENT_PULSE_WIDTH, msec)
    AAIR_VVIR.AAI_ATRIAL_PACING -> AAIR_VVIR.AAI_ARP_STATE : after(ATR_PULSE_WIDTH, msec)
  state DOOR
    state DOOR_ATR_CHARGE
      entry:
      FRONTEND_CTRL = true;
      %Charge C22
      ATR_PACE_CTRL=false;
      VENT_PACE_CTRL=false;
      PACE_CHARGE_CTRL=true;
      %Discharge C21 - discharging blocking capacitor
      PACE_GND_CTRL=true;
      ATR_GND_CTRL=true;
      VENT_GND_CTRL=false;
      LED_RED = false;
      PACING_REF_PWM = VENT_AMPLITUDE;
    state DOOR_VENT_PACING
      entry:
      FRONTEND_CTRL = false;
      PACE_CHARGE_CTRL=false;
      PACE_GND_CTRL=true;
      ATR_PACE_CTRL=false;
      ATR_GND_CTRL=false;
      VENT_GND_CTRL=false;
      VENT_PACE_CTRL=true;
      LED_GREEN = true;
      %% Green LED will turn on
    state DOOR_VENT_CHARGE
      entry:
      FRONTEND_CTRL = true;
      %Charge C22
      VENT_PACE_CTRL=false;
      ATR_PACE_CTRL=false;
      PACE_CHARGE_CTRL=true;
      %Discharge C21
      PACE_GND_CTRL=true;
      ATR_GND_CTRL=false;
      VENT_GND_CTRL=true;
      LED_GREEN = false;
      PACING_REF_PWM = ATR_AMPLITUDE;
    state DOOR_ATR_PACING
      entry:
      FRONTEND_CTRL = false;
      PACE_CHARGE_CTRL=false;
      PACE_GND_CTRL=true;
      ATR_PACE_CTRL=true;
      ATR_GND_CTRL=false;
      VENT_GND_CTRL=false;
      VENT_PACE_CTRL=false;
      LED_RED= true;
      %% RED LED will turn on
      %% Rate adaptive mode accounts for the adaptive period
    DOOR_ATR_CHARGE -> DOOR_VENT_PACING : after(AV_DELAY - ATR_PULSE_WIDTH,msec)
    DOOR_VENT_PACING -> DOOR_VENT_CHARGE : after(VENT_PULSE_WIDTH,msec)
    DOOR_ATR_PACING -> DOOR_ATR_CHARGE : after(ATR_PULSE_WIDTH,msec)
    (default) -> DOOR_VENT_CHARGE
    DOOR_VENT_CHARGE -> DOOR_ATR_PACING [order 1] : after(Adaptive_Period - AV_DELAY - VENT_PULSE_WIDTH,msec)
    DOOR_VENT_CHARGE -> DOOR [order 2] : [MODE ~=9]
  note: 7 is AAIR
      | 8 is VVIR
  note: 9 is DOOR
  state Init
    entry:
    ATR_PACE_CTRL=false;
    VENT_PACE_CTRL=false;
    PACE_CHARGE_CTRL=false;
    PACE_GND_CTRL=false;
    ATR_GND_CTRL=false;
    Z_ATR_CTRL =false;
    Z_VENT_CTRL = false;
    VENT_GND_CTRL=false;
    LED_RED = false;
    LED_GREEN = false;
    %Initalizations for all harware outputs
  state AOOR_VOOR
    state AOOR_CHARGE
      entry:
      FRONTEND_CTRL = true;
      ATR_PACE_CTRL=false;
      VENT_PACE_CTRL=false;
      PACE_CHARGE_CTRL=true;
      %Discharge C21
      PACE_GND_CTRL=true;
      ATR_GND_CTRL=true;
      VENT_GND_CTRL=false;
      LED_RED = false;
      PACING_REF_PWM = ATR_AMPLITUDE;
      %% Initially pulse is not sent and only sent after the first interval
      % 0 when (lower rate limit - atr pulse width)
      % 1 when (atr_pulse width)
      %% RED LED is turned off
    state VOOR_CHARGE
      entry:
      FRONTEND_CTRL = true;
      VENT_PACE_CTRL=false;
      ATR_PACE_CTRL=false;
      PACE_CHARGE_CTRL=true;
      %Discharge C21
      PACE_GND_CTRL=true;
      ATR_GND_CTRL=false;
      VENT_GND_CTRL=true;
      LED_GREEN = false;
      PACING_REF_PWM = VENT_AMPLITUDE;
      %% Initially pulse is not sent and only sent after the first interval
      % 0 when (lower rate limit - atr pulse width)
      % 1 when (atr_pulse width)
      %% GREEN LED is turned off
    state AOOR_DISCHARGE
      entry:
      FRONTEND_CTRL = false;
      PACE_CHARGE_CTRL=false;
      PACE_GND_CTRL=true;
      ATR_PACE_CTRL=true;
      ATR_GND_CTRL=false;
      VENT_GND_CTRL=false;
      VENT_PACE_CTRL=false;
      LED_RED= true;
      %% State when the pulse is sent and only for the ATR_PULSE_WIDTH
      %% RED LED will turn on
    state VOOR_DISCHARGE
      entry:
      FRONTEND_CTRL = false;
      PACE_CHARGE_CTRL=false;
      PACE_GND_CTRL=true;
      ATR_PACE_CTRL=false;
      ATR_GND_CTRL=false;
      VENT_GND_CTRL=false;
      VENT_PACE_CTRL=true;
      LED_GREEN = true;
      %% State when the pulse is sent and only for the ATR_PULSE_WIDTH
      %% Green LED will turn on
    AOOR_CHARGE -> AOOR_VOOR [order 2] : [MODE ~= 5]
    VOOR_CHARGE -> AOOR_VOOR [order 2] : [MODE ~=6]
    (default) -> (junction 147)
    (junction 147) -> AOOR_CHARGE [order 1] : [MODE == 5]
    (junction 147) -> VOOR_CHARGE [order 2]
    VOOR_CHARGE -> VOOR_DISCHARGE [order 1] : after(Adaptive_Period - VENT_PULSE_WIDTH,msec)
    VOOR_DISCHARGE -> VOOR_CHARGE : after(VENT_PULSE_WIDTH,msec)
    AOOR_CHARGE -> AOOR_DISCHARGE [order 1] : after(Adaptive_Period - ATR_PULSE_WIDTH,msec)
    AOOR_DISCHARGE -> AOOR_CHARGE : after(ATR_PULSE_WIDTH,msec)
  state DOO
    state DOO_VENT_CHARGE
      entry:
      FRONTEND_CTRL = true;
      %Charge C22
      ATR_PACE_CTRL=false;
      VENT_PACE_CTRL=false;
      PACE_CHARGE_CTRL=true;
      %Discharge C21 - discharging blocking capacitor
      PACE_GND_CTRL=true;
      ATR_GND_CTRL=true;
      VENT_GND_CTRL=false;
      LED_RED = false;
      PACING_REF_PWM = VENT_AMPLITUDE;
      %% Pacing amplitude is set to ventricle
    state DOO_VENT_PACING
      entry:
      FRONTEND_CTRL = true;
      PACE_CHARGE_CTRL=false;
      PACE_GND_CTRL=true;
      ATR_PACE_CTRL=false;
      ATR_GND_CTRL=false;
      VENT_GND_CTRL=false;
      VENT_PACE_CTRL=true;
      LED_GREEN = true;
      %% Green LED will turn on, Ventricle paces
    state DOO_ATR_CHARGE1
      entry:
      FRONTEND_CTRL = false;
      %Charge C22
      VENT_PACE_CTRL=false;
      ATR_PACE_CTRL=false;
      PACE_CHARGE_CTRL=true;
      %Discharge C21
      PACE_GND_CTRL=true;
      ATR_GND_CTRL=false;
      VENT_GND_CTRL=true;
      LED_GREEN = false;
      PACING_REF_PWM = ATR_AMPLITUDE;
      %% Pacing amplitude is set to atrium
    state DOO_ATR_PACING
      entry:
      FRONTEND_CTRL = false;
      PACE_CHARGE_CTRL=false;
      PACE_GND_CTRL=true;
      ATR_PACE_CTRL=true;
      ATR_GND_CTRL=false;
      VENT_GND_CTRL=false;
      VENT_PACE_CTRL=false;
      LED_RED= true;
      %% RED LED will turn on, Atrium paces
    DOO_VENT_CHARGE -> DOO_VENT_PACING : after(AV_DELAY - ATR_PULSE_WIDTH,msec)
    DOO_VENT_PACING -> DOO_ATR_CHARGE1 : after(VENT_PULSE_WIDTH,msec)
    DOO_ATR_PACING -> DOO_VENT_CHARGE : after(ATR_PULSE_WIDTH,msec)
    (default) -> DOO_ATR_CHARGE1
    DOO_ATR_CHARGE1 -> DOO_ATR_PACING [order 2] : after(Lower_Rate_Period - AV_DELAY - VENT_PULSE_WIDTH,msec)
    DOO_ATR_CHARGE1 -> DOO [order 1] : [MODE ~= 4]
  note: 5 is AOOR
      | 6 is VOOR
  note: 4 is DOO
  note: 2 is AAI
      | 3 is VVI
  note: 0 is AOO
      | 1 is VOO
  state AOO_VOO
    state VOO_CHARGE
      entry:
      FRONTEND_CTRL = true;
      VENT_PACE_CTRL=false;
      ATR_PACE_CTRL=false;
      PACE_CHARGE_CTRL=true;
      %Discharge C21
      PACE_GND_CTRL=true;
      ATR_GND_CTRL=false;
      PACING_REF_PWM = VENT_AMPLITUDE;
      VENT_GND_CTRL=true;
      LED_GREEN = false;
      %% Initially pulse is not sent and only sent after the first interval
      % 0 when (lower rate limit - atr pulse width)
      % 1 when (atr_pulse width)
      %% GREEN LED is turned off
      %When the mode is changed from 1, it will exit this state and enter
      %    the initial state
    state AOO_CHARGE
      entry:
      FRONTEND_CTRL = true;
      ATR_PACE_CTRL=false;
      VENT_PACE_CTRL=false;
      PACE_CHARGE_CTRL=true;
      %Discharge C21
      PACE_GND_CTRL=true;
      ATR_GND_CTRL=true;
      PACING_REF_PWM = ATR_AMPLITUDE;
      VENT_GND_CTRL=false;
      LED_RED = false;
      %% Initially pulse is not sent and only sent after the first interval
      % 0 when (lower rate limit - atr pulse width)
      % 1 when (atr_pulse width)
      %% RED LED is turned off
      %When the mode is changed from 0, it will exit this state and enter
      %    the initial state
    state AOO_DISCHARGE
      entry:
      FRONTEND_CTRL = false;
      PACE_CHARGE_CTRL=false;
      PACE_GND_CTRL=true;
      ATR_PACE_CTRL=true;
      ATR_GND_CTRL=false;
      VENT_GND_CTRL=false;
      VENT_PACE_CTRL=false;
      LED_RED= true;
      %% State when the pulse is sent and only for the ATR_PULSE_WIDTH
      %% RED LED will turn on
    state VOO_DISCHARGE
      entry:
      FRONTEND_CTRL = false;
      PACE_CHARGE_CTRL=false;
      PACE_GND_CTRL=true;
      ATR_PACE_CTRL=false;
      ATR_GND_CTRL=false;
      VENT_GND_CTRL=false;
      VENT_PACE_CTRL=true;
      LED_GREEN = true;
      %% State when the pulse is sent and only for the ATR_PULSE_WIDTH
      %% Green LED will turn on
    AOO_CHARGE -> AOO_VOO [order 2] : [MODE ~=0]
    VOO_CHARGE -> AOO_VOO [order 2] : [MODE ~=1]
    (default) -> (junction 10)
    (junction 10) -> VOO_CHARGE [order 2]
    (junction 10) -> AOO_CHARGE [order 1] : [MODE == 0]
    AOO_CHARGE -> AOO_DISCHARGE [order 1] : after(Lower_Rate_Period - ATR_PULSE_WIDTH,msec)
    AOO_DISCHARGE -> AOO_CHARGE : after(ATR_PULSE_WIDTH,msec)
    VOO_CHARGE -> VOO_DISCHARGE [order 1] : after(Lower_Rate_Period- VENT_PULSE_WIDTH,msec)
    VOO_DISCHARGE -> VOO_CHARGE : after(VENT_PULSE_WIDTH,msec)
  state AAI_VVI
    state AAI_CHARGING
      entry:
      FRONTEND_CTRL = true;
      PACE_GND_CTRL = true;
      VENT_PACE_CTRL=false;
      ATR_PACE_CTRL=false;
      PACE_CHARGE_CTRL=true;
      ATR_GND_CTRL=false;
      VENT_GND_CTRL=true;
      LED_RED = false;
      PACING_REF_PWM = ATR_AMPLITUDE;
      % charging and discharging the capacitors
      % setting the pacing pwm to Atrium Amplitude
    state VVI_CHARGING
      entry:
      FRONTEND_CTRL = true;
      PACE_GND_CTRL = true;
      VENT_PACE_CTRL=false;
      ATR_PACE_CTRL=false;
      PACE_CHARGE_CTRL=true;
      ATR_GND_CTRL=false;
      VENT_GND_CTRL=true;
      LED_GREEN = false;
      PACING_REF_PWM = VENT_AMPLITUDE;
      % charging and discharging the capacitors
      % setting the pacing pwm to Ventricle Amplitude
    state VVI_ATRIAL_PACING
      entry:
      FRONTEND_CTRL = false;
      PACE_GND_CTRL = true;
      VENT_PACE_CTRL=true;
      ATR_PACE_CTRL=false;
      PACE_CHARGE_CTRL=false;
      ATR_GND_CTRL=false;
      VENT_GND_CTRL=false;
      LED_GREEN = true;
      %pacemaker will respond by sending a signal
    state AAI_ATRIAL_PACING
      entry:
      FRONTEND_CTRL = false;
      PACE_GND_CTRL = true;
      VENT_PACE_CTRL=false;
      ATR_PACE_CTRL=true;
      PACE_CHARGE_CTRL=false;
      ATR_GND_CTRL=false;
      VENT_GND_CTRL=false;
      LED_RED = true;
      %pacemaker will respond by sending a signal
    state AAI_ARP_STATE
      entry:
      PACE_GND_CTRL = true;
      VENT_PACE_CTRL=false;
      ATR_PACE_CTRL=false;
      PACE_CHARGE_CTRL=true;
      ATR_GND_CTRL=true;
      VENT_GND_CTRL=false;
      LED_RED= false;
      %enters this state when a atrial signal is detected
    state VVI_VRP_STATE
      entry:
      PACE_GND_CTRL = true;
      VENT_PACE_CTRL=false;
      ATR_PACE_CTRL=false;
      PACE_CHARGE_CTRL=true;
      ATR_GND_CTRL=false;
      VENT_GND_CTRL=true;
      LED_GREEN = false;
      PACING_REF_PWM = VENT_AMPLITUDE;
      %enters this state when a ventricle signal is detected
    AAI_CHARGING -> AAI_VVI [order 2] : [MODE ~=2]
    AAI_VVI.VVI_CHARGING -> AAI_VVI [order 2] : [MODE ~=3]
    (junction 21) -> AAI_CHARGING [order 1] : [MODE == 2]
    (default) -> (junction 21)
    (junction 21) -> AAI_VVI.VVI_CHARGING [order 2]
    AAI_VVI.VVI_CHARGING -> AAI_VVI.VVI_ATRIAL_PACING [order 1] : after(Lower_Rate_Period - VENT_PULSE_WIDTH-VRP, msec)
    AAI_CHARGING -> AAI_VVI.AAI_ATRIAL_PACING [order 1] : after((Lower_Rate_Period) - ATR_PULSE_WIDTH - ARP, msec)
    AAI_VVI.VVI_VRP_STATE -> AAI_VVI.VVI_CHARGING : after(VRP, msec)
    AAI_VVI.VVI_CHARGING -> AAI_VVI.VVI_VRP_STATE [order 3] : [VENT_CMP_DETECT == true]
    AAI_CHARGING -> AAI_VVI.AAI_ARP_STATE [order 3] : [ATR_CMP_DETECT == true]
    AAI_VVI.AAI_ARP_STATE -> AAI_CHARGING : after(ARP, msec)
    AAI_VVI.VVI_ATRIAL_PACING -> AAI_VVI.VVI_VRP_STATE : after(VENT_PULSE_WIDTH, msec)
    AAI_VVI.AAI_ATRIAL_PACING -> AAI_VVI.AAI_ARP_STATE : after(ATR_PULSE_WIDTH, msec)
  AAIR_VVIR -> Init : [MODE ~= 7 && MODE ~= 8]
  Init -> DOOR [order 6] : [MODE == 9]
  (default) -> Init
  DOOR -> Init : [MODE ~= 9]
  Init -> AAIR_VVIR [order 5] : [MODE == 7 || MODE == 8]
  Init -> DOO [order 2] : [MODE == 4]
  AOOR_VOOR -> Init : [MODE ~= 5 && MODE ~= 6]
  DOO -> Init : [MODE ~= 4]
  Init -> AOOR_VOOR [order 4] : [MODE == 5 || MODE == 6]
  AOO_VOO -> Init : [MODE ~= 0 && MODE ~=1]
  Init -> AOO_VOO [order 1] : [MODE == 0 || MODE ==1]
  Init -> Init [order 7] : [Lower_Rate_Limit<=Upper_Rate_Limit]
  AAI_VVI -> Init : [MODE ~= 2 && MODE ~=3]
  Init -> AAI_VVI [order 3] : [MODE == 2 || MODE ==3]
  data: Upper_Rate_Limit input; Adaptive_Period input; ATR_PULSE_WIDTH input uint16; VRP input uint16; ARP input uint16; VENT_PULSE_WIDTH input uint16; MODE input uint16; ATR_CMP_DETECT input boolean; VENT_AMPLITUDE input single; ATR_AMPLITUDE input single; AV_DELAY input; Lower_Rate_Period input double; LED_RED output boolean; PACE_CHARGE_CTRL output boolean; VENT_PACE_CTRL output boolean; VENT_GND_CTRL output boolean; PACE_GND_CTRL output boolean; ATR_PACE_CTRL output boolean; FRONTEND_CTRL output boolean; ATR_GND_CTRL output boolean; Z_VENT_CTRL output boolean; Z_ATR_CTRL output boolean; LED_GREEN output boolean; VENT_CMP_DETECT input boolean; PACING_REF_PWM output; Lower_Rate_Limit input

== stateflow chart Group10_Pacemaker_FinalSimulink/COM_IN ==
  note: MODE
      | Atrial_Pulse_Width
      | Ventricle_Pulse_Width
      | Lower_Rate_Limit
      | Upper_Rate_Limit**
      | VRP
      | ARP
      | AV_Delay
      | Reaction_Time
      | Recovery_Time
      | Response_Factor
      |
      | float
      | Atrial_Sensing
      | Ventricle_Sensing
      | Atrial_Amplitude
      | Ventricle_Amplitude
      | Activity_Threshold
  state Params
    entry:
    MODE = typecast(rxdata(3:4),'uint16')
    Lower_Rate_Limit = typecast(rxdata(5:6),'uint16')
    Upper_Rate_Limit =typecast(rxdata(7:8),'uint16')
    Atrial_Amplitude =  typecast(rxdata(9:12),'single')
    Atrial_Pulse_Width = typecast(rxdata(13:14),'uint16')
    Ventricle_Amplitude =  typecast(rxdata(15:18),'single')
    Ventricle_Pulse_Width =typecast(rxdata(19:20),'uint16')
    VRP = typecast(rxdata(21:22),'uint16')
    ARP=typecast(rxdata(23:24),'uint16')
    AV_Delay = typecast(rxdata(25:26),'uint16')
    Reaction_Time = typecast(rxdata(27:28),'uint16')
    Recovery_Time =typecast(rxdata(29:30),'uint16')
    Activity_Threshold = typecast(rxdata(31:38),'double')
    Max_Sensor_Rate = typecast(rxdata(39:40),'uint16')
    Rate_Smoothing =typecast(rxdata(41:42),'uint16')
    Atrial_Sensing = typecast(rxdata(43:46),'single')
    Ventricle_Sensing = typecast(rxdata(47:50),'single')
    Response_Factor = typecast(rxdata(51:52),'uint16')
  state Init_Parameters
    entry:
    Ventricle_Pulse_Width = 1
    Atrial_Pulse_Width =5
    VRP = 250
    ARP= 250
    MODE =10
    Lower_Rate_Limit = 60
    Upper_Rate_Limit =120
    Atrial_Sensing  = 5
    Ventricle_Sensing = 5
    Atrial_Amplitude = 5
    Ventricle_Amplitude = 5
    Reaction_Time = 30
    AV_Delay = 100
    Response_Factor=8
    Recovery_Time =5
    Max_Sensor_Rate = 120
    Activity_Threshold = 0.2
    Rate_Smoothing = 0
    %Initial Parameters that the pacemaker will be set to
  state STANDBY
    LED_BLUE = false
  state ECHO_PARAM
    entry:
    send_parameters();
    LED_BLUE = true
    %this calls the send_parameters function
  Params -> STANDBY
  (default) -> Init_Parameters
  (junction 10) -> Params [order 1] : [rxdata(2) ==hex2dec('12')]
  (junction 9) -> STANDBY [order 2]
  STANDBY -> (junction 9) : [status == 0]
  (junction 9) -> (junction 10) [order 1] : [rxdata(1) == hex2dec('16') ]
  Init_Parameters -> STANDBY
  (junction 10) -> ECHO_PARAM [order 2] : [rxdata(2) == hex2dec('16')]
  ECHO_PARAM -> STANDBY
  data: LED_BLUE output; Atrial_Pulse_Width output uint16; MODE output uint16; Lower_Rate_Limit output uint16; Ventricle_Sensing output single; Atrial_Amplitude output single; Ventricle_Amplitude output single; Reaction_Time output uint16; Upper_Rate_Limit output uint16; Atrial_Sensing output single; ARP output uint16; AV_Delay output uint16; Response_Factor output uint16; Recovery_Time output uint16; Max_Sensor_Rate output uint16; Ventricle_Pulse_Width output uint16; rxdata input uint8; status input uint8; VRP output uint16; Activity_Threshold output double; Rate_Smoothing output uint16

== matlab function Group10_Pacemaker_FinalSimulink/Input_Conversion/MATLAB Function1 ==
  data: u input; y output
function y = fcn(u)

y = u./5.*100;

== matlab function Group10_Pacemaker_FinalSimulink/Input_Conversion/MATLAB Function2 ==
  data: u input; y output
function y = fcn(u)

y = u./5.*100;
